simulink model "step4-c"  (R2020b)
settings: Solver=VariableStepAuto  StartTime=0.0  StopTime=15  RelTol=1e-3
libraries: dspsrcs4 x1, dspadpt3 x1
settings Model: Creator=Borma  LastModifiedBy=Borma

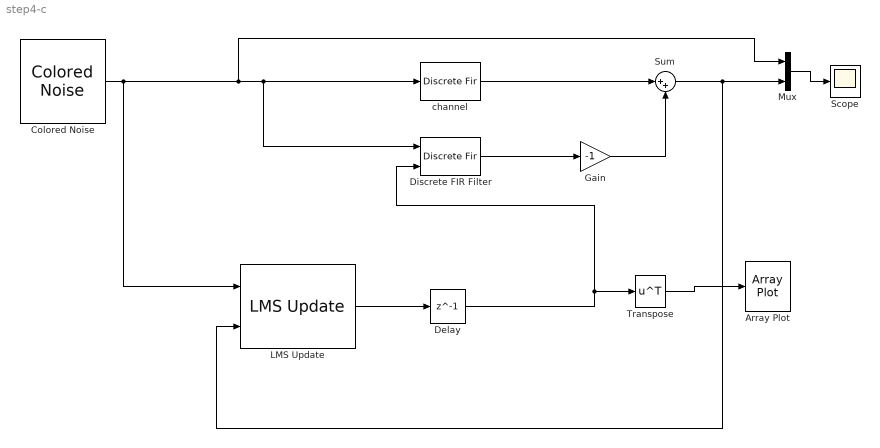
== system step4-c ==
  Array Plot : ArrayPlot
  Colored Noise : dspsrcs4/Colored Noise  Color=pink  InverseFrequencyPower=1  BoundedOutput=off  NumChannels=1  OutputDataType=double  SamplesPerFrame=1  SampleTime=1/4000  RandomStream=mt19937ar with seed  Seed=67  SimulateUsing=Interpreted execution
      settings: SourceProductBaseCode=DS
  Delay : Delay  DelayLength=1  InitialCondition=0
  Discrete FIR Filter : DiscreteFir  CoefSource=Input port  InputProcessing=Columns as channels (frame based)
      settings: InputPortMap=u0,u1
  Gain : Gain  Gain=-1
  LMS Update : dspadpt3/LMS Update  Method=Normalized LMS  Length=24  StepSizeSource=Property  StepSize=0.01  LeakageFactor=1.0  InitialConditions=0  EnableAdaptInput=off  EnableResetInput=off  SimulateUsing=Code generation
      settings: SourceProductBaseCode=DS
  Mux : Mux  Inputs=2
  Scope : Scope
  Sum : Sum  Inputs=|++
  Transpose : Math  Operator=transpose  SaturateOnIntegerOverflow=on
  channel : DiscreteFir  Coefficients=[0.5 0.1 0.2 0.4 0 0 -0.125 0.3 0.5 0 0.075 -0.25 -0.4]
  wires:
  LMS Update/1 -> Delay/1
  Delay/1 -> Transpose/1, Discrete FIR Filter/2
  Colored Noise/1 -> LMS Update/1, Mux/1, Discrete FIR Filter/1, channel/1
  Discrete FIR Filter/1 -> Gain/1
  Sum/1 -> LMS Update/2, Mux/2
  channel/1 -> Sum/1
  Mux/1 -> Scope/1
  Gain/1 -> Sum/2
  Transpose/1 -> Array Plot/1
